simulink model "OSMAAD003_LanderModelV2"  (R2018a)
settings: Solver=ode4  StartTime=0.0  StopTime=45  FixedStep=0.001  RelTol=1e-3
values from neighbouring files (symbols this model uses):
  K = lqr (A_lin,B_lin,Q,R)    [OSMAAD003_setup_controller.m]
  K_180 = lqr(A_lin,B_lin,Q,R)    [OSMAAD003_setup_controller.m]
libraries: simulink x1
settings Model: Creator=KNMALE002  LastModifiedBy=aadam
settings DataIOCC: SaveOutput=off  SignalLogging=off  DSMLogging=off
settings DebuggingCC: LibraryContextMissingDiagnostic=warning
settings SFSimCC: SimUseLocalCustomCode=on
settings RTWCC: RTWUseLocalCustomCode=on

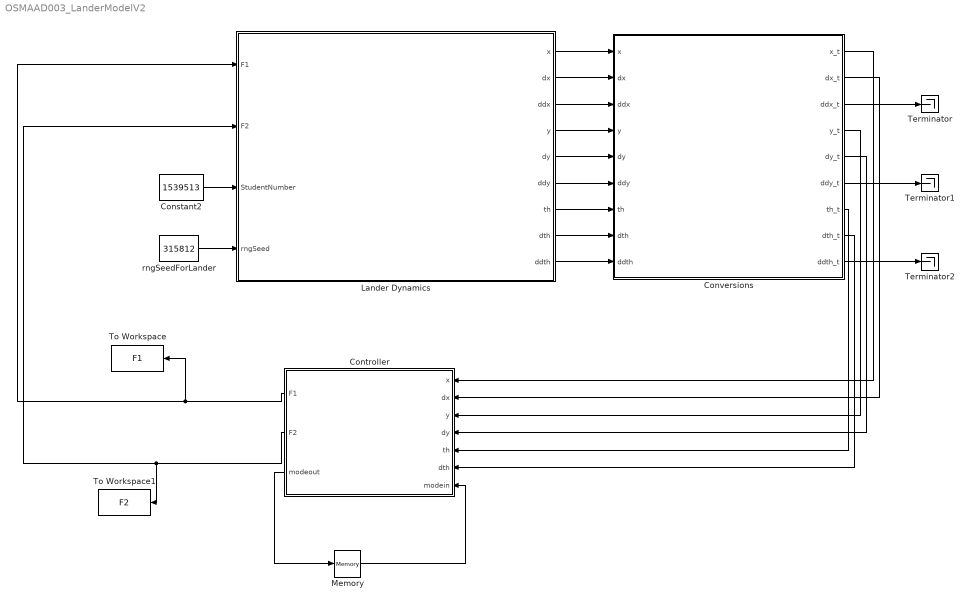
== system OSMAAD003_LanderModelV2 ==
  Constant2 : Constant  Value=1539513
  Controller : MATLAB Function  TreatAsAtomicUnit=on
  Conversions : Subsystem
  Lander Dynamics : Subsystem  TreatAsAtomicUnit=on  mask{Value=1}
      mask prompts: Value "Enter mode (1, 2 or 3)"
      mask TypeOptions Value: ModeVar/Value
      mask Display: image('lander.jpg');
  Memory : Memory  InheritSampleTime=on  LinearizeAsDelay=on
  Terminator : Terminator
  Terminator1 : Terminator
  Terminator2 : Terminator
  To Workspace : ToWorkspace  VariableName=F1  SaveFormat=Structure With Time  SampleTime=-1
  To Workspace1 : ToWorkspace  VariableName=F2  SaveFormat=Structure With Time  SampleTime=-1
  rngSeedForLander : Constant  Value=315812
  wires:
  Constant2/1 -> Lander Dynamics/3(StudentNumber)
  Lander Dynamics/2(dx) -> Conversions/2(dx)
  Lander Dynamics/3(ddx) -> Conversions/3(ddx)
  Lander Dynamics/6(ddy) -> Conversions/6(ddy)
  Lander Dynamics/9(ddth) -> Conversions/9(ddth)
  rngSeedForLander/1 -> Lander Dynamics/4(rngSeed)
  Lander Dynamics/1(x) -> Conversions/1(x)
  Lander Dynamics/4(y) -> Conversions/4(y)
  Lander Dynamics/5(dy) -> Conversions/5(dy)
  Lander Dynamics/7(th) -> Conversions/7(th)
  Lander Dynamics/8(dth) -> Conversions/8(dth)
  Conversions/1(x_t) -> Controller/1(x)
  Conversions/2(dx_t) -> Controller/2(dx)
  Conversions/4(y_t) -> Controller/3(y)
  Conversions/5(dy_t) -> Controller/4(dy)
  Conversions/8(dth_t) -> Controller/6(dth)
  Conversions/3(ddx_t) -> Terminator/1
  Conversions/6(ddy_t) -> Terminator1/1
  Conversions/9(ddth_t) -> Terminator2/1
  Controller/1(F1) -> To Workspace/1, Lander Dynamics/1(F1)
  Controller/2(F2) -> To Workspace1/1, Lander Dynamics/2(F2)
  Conversions/7(th_t) -> Controller/5(th)
  Controller/3(modeout) -> Memory/1
  Memory/1 -> Controller/7(modein)

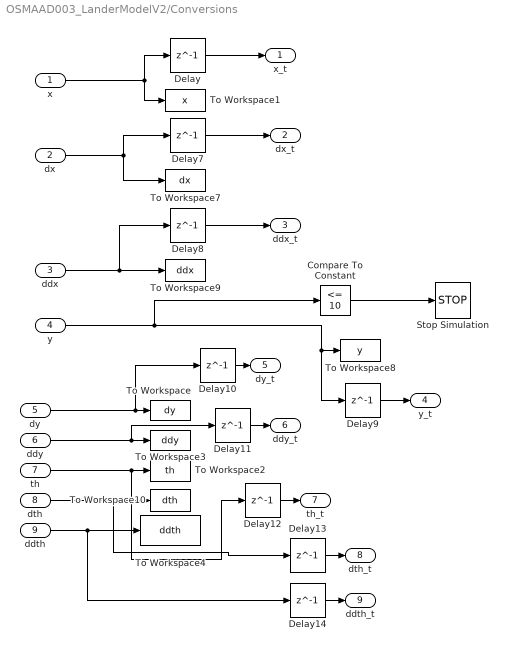
== system OSMAAD003_LanderModelV2/Conversions ==
  x : Inport
  dx : Inport  Port=2
  ddx : Inport  Port=3
  y : Inport  Port=4
  dy : Inport  Port=5
  ddy : Inport  Port=6
  th : Inport  Port=7
  dth : Inport  Port=8
  ddth : Inport  Port=9
  Compare To Constant : simulink/Logic and Bit Operations/Compare To Constant  relop=<=  const=10  OutDataTypeStr=boolean
  Delay{,7..14} (9 alike) : Delay  DelayLength=1
  Stop Simulation : Stop
  To Workspace : ToWorkspace  VariableName=dy  SaveFormat=Structure With Time  SampleTime=-1
  To Workspace1 : ToWorkspace  VariableName=x  SaveFormat=Structure With Time  SampleTime=-1
  To Workspace10 : ToWorkspace  VariableName=dth  SaveFormat=Structure With Time  SampleTime=-1
  To Workspace2 : ToWorkspace  VariableName=th  SaveFormat=Structure With Time  SampleTime=-1
  To Workspace3 : ToWorkspace  VariableName=ddy  SaveFormat=Structure With Time  SampleTime=-1
  To Workspace4 : ToWorkspace  VariableName=ddth  SaveFormat=Structure With Time  SampleTime=-1
  To Workspace7 : ToWorkspace  VariableName=dx  SaveFormat=Structure With Time  SampleTime=-1
  To Workspace8 : ToWorkspace  VariableName=y  SaveFormat=Structure With Time  SampleTime=-1
  To Workspace9 : ToWorkspace  VariableName=ddx  SaveFormat=Structure With Time  SampleTime=-1
  x_t : Outport
  dx_t : Outport  Port=2
  ddx_t : Outport  Port=3
  y_t : Outport  Port=4
  dy_t : Outport  Port=5
  ddy_t : Outport  Port=6
  th_t : Outport  Port=7
  dth_t : Outport  Port=8
  ddth_t : Outport  Port=9
  wires:
  Delay13/1 -> dth_t/1
  Delay11/1 -> ddy_t/1
  Delay7/1 -> dx_t/1
  ddx/1 -> Delay8/1, To Workspace9/1
  Compare To Constant/1 -> Stop Simulation/1
  ddy/1 -> Delay11/1, To Workspace3/1
  th/1 -> Delay12/1, To Workspace2/1
  Delay14/1 -> ddth_t/1
  x/1 -> Delay/1, To Workspace1/1
  ddth/1 -> Delay14/1, To Workspace4/1
  dth/1 -> Delay13/1, To Workspace10/1
  Delay12/1 -> th_t/1
  y/1 -> Delay9/1, To Workspace8/1, Compare To Constant/1
  Delay8/1 -> ddx_t/1
  dy/1 -> Delay10/1, To Workspace/1
  Delay/1 -> x_t/1
  dx/1 -> To Workspace7/1, Delay7/1
  Delay10/1 -> dy_t/1
  Delay9/1 -> y_t/1

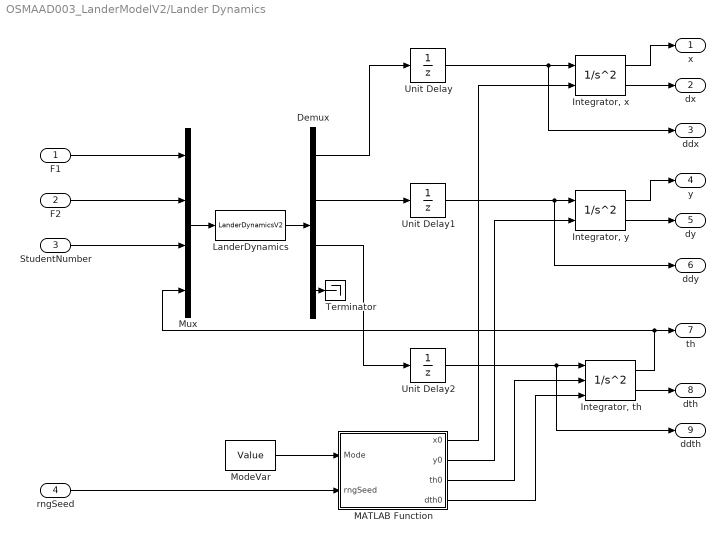
== system OSMAAD003_LanderModelV2/Lander Dynamics ==
  F1 : Inport
  F2 : Inport  Port=2
  StudentNumber : Inport  Port=3
  rngSeed : Inport  Port=4
  Demux : Demux
  "Integrator, th" : SecondOrderIntegrator  ICSourceX=external  ICX=th0  ICSourceDXDT=external  ICDXDT=dth0
  "Integrator, x" : SecondOrderIntegrator  ICSourceX=external  ICX=x0
  "Integrator, y" : SecondOrderIntegrator  ICSourceX=external  ICX=y0
  LanderDynamics : MATLABFcn  MATLABFcn=LanderDynamicsV2  Output1D=off
  MATLAB Function : MATLAB Function  TreatAsAtomicUnit=on
  ModeVar : Constant  Value=Value
  Mux : Mux
  Terminator : Terminator
  Unit Delay : UnitDelay  SampleTime=-1
  Unit Delay1 : UnitDelay  SampleTime=-1
  Unit Delay2 : UnitDelay  SampleTime=-1
  x : Outport  PortDimensions=1
  dx : Outport  Port=2  PortDimensions=1
  ddx : Outport  Port=3  PortDimensions=1
  y : Outport  Port=4  PortDimensions=1
  dy : Outport  Port=5  PortDimensions=1
  ddy : Outport  Port=6  PortDimensions=1
  th : Outport  Port=7  PortDimensions=1
  dth : Outport  Port=8  PortDimensions=1
  ddth : Outport  Port=9  PortDimensions=1
  wires:
  "Integrator, th"/1 -> Mux/4, th/1
  Unit Delay/1 -> ddx/1, "Integrator, x"/1
  Unit Delay1/1 -> ddy/1, "Integrator, y"/1
  Unit Delay2/1 -> ddth/1, "Integrator, th"/1
  "Integrator, x"/1 -> x/1
  "Integrator, x"/2 -> dx/1
  "Integrator, y"/2 -> dy/1
  "Integrator, y"/1 -> y/1
  "Integrator, th"/2 -> dth/1
  Mux/1 -> LanderDynamics/1
  LanderDynamics/1 -> Demux/1
  rngSeed/1 -> MATLAB Function/2(rngSeed)
  ModeVar/1 -> MATLAB Function/1(Mode)
  MATLAB Function/1(x0) -> "Integrator, x"/2
  MATLAB Function/2(y0) -> "Integrator, y"/2
  MATLAB Function/3(th0) -> "Integrator, th"/2
  MATLAB Function/4(dth0) -> "Integrator, th"/3
  F1/1 -> Mux/1
  F2/1 -> Mux/2
  StudentNumber/1 -> Mux/3
  Demux/1 -> Unit Delay/1
  Demux/2 -> Unit Delay1/1
  Demux/3 -> Unit Delay2/1
  Demux/4 -> Terminator/1

== matlab function OSMAAD003_LanderModelV2/Lander Dynamics/MATLAB Function ==
  data: x0 output; y0 output; th0 output; dth0 output; Mode input; rngSeed input
function [x0, y0, th0, dth0] = fcn(Mode, rngSeed)
% for reference, 0.5rad = 28 deg
rng(rngSeed);

if (Mode == 1)
    x0 = 0;
    y0 = 1000 + (rand(1)-0.5)*10;  % +- 5
    th0 = 0;
    dth0 = 0;
elseif (Mode == 2)
    x0 = 0;
    y0 = 1000 + (rand(1)-0.5)*100; % +- 50
    th0 = (rand(1)-0.5);           % +- 0.5
    dth0 = 0;
elseif (Mode == 3)
    x0 = 0;
    y0 = 1200 + randi([-300, 300]);
    th0 = pi + 2*(rand(1)-0.5);      % upside down, +- 0.5
    dth0 = 0.2*(rand(1)-0.5);        % +- 0.1 rad/sec
else
    disp('You entered the mode incorrectly. Make sure Mode = 1, 2 or 3')
    x0 = 0;
    y0 = 0;
    th0 = 0;
    dth0 = 0;
end

== matlab function OSMAAD003_LanderModelV2/Controller ==
  data: x input; dx input; F1 output; F2 output; y input; dy input; th input; dth input; K parameter; K_180 parameter; modein input; modeout output
function [F1, F2, modeout] = fcn(x,dx,y,dy,th,dth,K, K_180,modein)
y = y-10;

modeout = modein;

if (abs(th)>1.3)
    modeout = 1;
end

if(modeout==1)
    u = -K_180*[th;dth];
    F1 = u(1);
    F2 =u(2);
    if(abs(th)<0.09)
        modeout = 0;
    end
else
    u = -K*[x;dx;y;dy;th;dth];
    F1 = 4000*9.3/2 +u(1);
    F2 = 4000*9.3/2 +u(2);
    modeout =0;
end

if(F1<0)
    F1=0;
end
if(F2<0)
    F2=0;
end


if(F1>74400)
    F1=74400;
end

if(F2>74400)
    F2=74400;
end


end
